simulink model "ALL_JP360_DBW_V6_5_1103"  (R2022a)
settings: Solver=FixedStepAuto  StartTime=0.0  StopTime=inf  FixedStep=0.01  RelTol=1e-3  EnableMultiTasking=on
model workspace (MAT data in the model file):
  g = 9.8
undefined symbols (not defined in the file or in its folder): canChannel, delta_v_p, IPM_Line_C0, IPM_Line_C1, IPM_Line_C2, IPM_Line_C3, M, M_p, MRR_ObjDistX, MRR_ObjDistY, MRR_ObjFusionCamID, MRR_ObjFusionSig, MRR_ObjID, MRR_ObjRelVelX, MRR_ObjRelVelY, MRR_ObjType, MRR_ObjUpdFlg, none, obj_vaild, untracktime, V, videoinput
libraries: canfdmsglib x230, canfdlib x76, slpidlib x24, simulink x18, dspstat3 x14, ctrlSharedLib x1, simulink_extras x1, imaqlib x1, realtime_pacer_lib x1, dspvision x1, visionsinks x1
(part 50 of 55)

== system ALL_JP360_DBW_V6_5_1103/button/ACCset/ACC_button ==
  Input : Inport
  SWM_ACCSwitch : Inport  Port=2
  SWM_ACCvSetPlus : Inport  Port=3
  SWM_ACCvSetMinus : Inport  Port=4
  set_speed_out : Inport  Port=5
  Add1 : Sum  Inputs=+-
  Add3 : Sum  Inputs=+-
  Add4 : Sum  Inputs=+-
  Chart1 : Stateflow chart  TreatAsAtomicUnit=on
      settings: RTWSystemCode=Reusable function
  Chart2 : Stateflow chart  TreatAsAtomicUnit=on
      settings: RTWSystemCode=Reusable function
  Data Store Read : DataStoreRead  DataStoreName=SpdSetValue  IndexOptions=Index vector (dialog)  Indices=1  OutputSizes=1
  Data Store Write2 : DataStoreWrite  DataStoreName=SpdSetValue  IndexOptions=Index vector (dialog)  Indices=1  OutputSizes=1
  Data Type Conversion : DataTypeConversion  OutDataTypeStr=uint8  SaturateOnIntegerOverflow=off  RndMeth=Floor
  Data Type Conversion1 : DataTypeConversion  OutDataTypeStr=single  SaturateOnIntegerOverflow=off  RndMeth=Floor
  Display : Display
  Memory{,1,7..8} (4 alike) : Memory
  OR3 : Logic  Operator=OR  Inputs=3  IconShape=distinctive  AllPortsSameDT=off  OutDataTypeStr=boolean
  Saturation : Saturate  UpperLimit=2  LowerLimit=0  OutDataTypeStr=int8
  Scope : Scope
  Subsystem1 : Subsystem  TreatAsAtomicUnit=on
      settings: MinAlgLoopOccurrences=on
  Subsystem2 : Subsystem  TreatAsAtomicUnit=on
      settings: MinAlgLoopOccurrences=on
  Subsystem3 : Subsystem  TreatAsAtomicUnit=on
      settings: MinAlgLoopOccurrences=on
  Subsystem4 : Subsystem  TreatAsAtomicUnit=on
      settings: MinAlgLoopOccurrences=on
  accsetv1 : Stateflow chart  TreatAsAtomicUnit=on
      settings: RTWSystemCode=Reusable function
  accsetv2 : Stateflow chart  TreatAsAtomicUnit=on
      settings: RTWSystemCode=Reusable function
  setvspeed : Outport
  SWM_ACCSwitchOut : Outport  Port=2
  wires:
  Subsystem3/1(Out1) -> Chart1/1(plus), Memory7/1, Add3/1
  Subsystem1/1(Out1) -> Memory8/1, Chart1/2(min), Add4/1
  [SWM_ACCvSetMinus] -> accsetv1/2(speed)
  SWM_ACCvSetPlus/1 -> [SWM_ACCvSetPlus]
  Memory7/1 -> Add3/2
  Chart1/1(a) -> Data Type Conversion/1, Display/1, Scope/1
  Add3/1 -> OR3/1
  SWM_ACCvSetMinus/1 -> [SWM_ACCvSetMinus]
  [SWM_ACCSwitch] -> Subsystem2/1(speedout)
  Input/1 -> [accsinp]
  Chart2/1(speedout) -> setvspeed/1
  SWM_ACCSwitch/1 -> [SWM_ACCSwitch]
  [SWM_ACCvSetPlus] -> accsetv2/2(speed)
  OR3/1 -> Chart1/Trigger
  Add4/1 -> OR3/2
  Memory8/1 -> Add4/2
  Subsystem2/1(Out1) -> Saturation/1
  Saturation/1 -> SWM_ACCSwitchOut/1  "SWM_ACCSwitchOut"
  [accstatus] -> accsetv1/1(accs)
  set_speed_out/1 -> Data Store Write2/1
  Memory1/1 -> Add1/2
  Data Store Read/1 -> Data Type Conversion1/1
  Add1/1 -> OR3/3
  [accsinp] -> Memory/1
  Memory/1 -> Subsystem4/1(speedout1)
  Subsystem4/1(Out1) -> [accstatus]
  accsetv2/1(speedout) -> Subsystem3/1(speedout)
  accsetv1/1(speedout) -> Subsystem1/1(speedout)
  [accstatus] -> accsetv2/1(accs)
  Data Type Conversion/1 -> Chart2/1(speed)
  Data Type Conversion1/1 -> Add1/1, Chart1/3(speed), Memory1/1

== system ALL_JP360_DBW_V6_5_1103/ACC_Control/ACC_FUNCTION/Subsystem2/ACC_model ==
  note: === Adaptive Cruise Control (ACC) autonomous system ===
      |
      |  - automatically controls the speed of the EGO vehicle,
      |  - is capable of assisting the driver to keep a safe distance
      |    from the preceding vehicle,
      |  - is controlling the engine throttle and brake pressure,
      |  - based on on-board, Technology Independent Sensors (TIS),
      |  - facilitates driving and partialy helps to prevent accidents.
  note: === ACC自适应巡航系统 ===
      |
      |  - 自动控制自车速度
      |  - 与前车保持安全距离
      |  - 自动控制刹车和油门防止碰撞
  note: 1/横摆角速度大于0.5°/s（可标定）时认为是过弯；
      | 2/弯道半径
  accstatus : Inport
  EGO_velocity_IC [m/s] : Inport  Port=2
  TIS1_range [m] : Inport  Port=3
  TIS1_rangedot [m/s] : Inport  Port=4
  HWT_dem [s] : Inport  Port=5
  Standstill_distance [m] : Inport  Port=6
  Des_speed[m/s] : Inport  Port=7
  obj_detacted_flag : Inport  Port=8
  abs_speed[m/s] : Inport  Port=9
  ax_esp[m/s2] : Inport  Port=10
  yaw_rate[deg/s] : Inport  Port=11
  steer_angle[deg] : Inport  Port=12
  ay_esp[m/s2] : Inport  Port=13
  IC_V_kph : Inport  Port=14
  CC_module : Subsystem  mask{DeltaV_Mul=5/3.6, Kp0=0.5, Kp1=0.01, Ki=0.005, Kd=0.05, Uplimit_acc=2, Uplimit_dec=-3}
      mask prompts: DeltaV_Mul "速度分段控制DeltaV_Mul"; Kp0 "速度误差大时Kp0"; Kp1 "速度误差小时Kp1"; Ki "定速巡航KI"; Kd "定速巡航Kd"; Uplimit_acc "定速巡航加速度上限Uplimit_acc"; Uplimit_dec "定速巡航减速度上线Uplimit_dec"
      mask DialogControl ParameterGroupVar Prompt: 参数
  Constant : Constant  Value=0  OutDataTypeStr=single
  Dead Zone : DeadZone  LowerValue=-1.2/57.3  UpperValue=1.2/57.3
  Gain3 : Gain  Gain=1/57.3
  Product : Product
  Rate transition from other signals1 : Subsystem  Commented=on
  Rate transition from EGO1 : Subsystem  Commented=on
  Rate transition from TIS2 : Subsystem  Commented=on
  Saturation1 : Saturate  UpperLimit=20/57.3  LowerLimit=-20/57.3
  Scope : Scope  NumInputPorts=2
  TIS1 ACC action : Subsystem
  calculate_slope : Subsystem
  curve agl : Subsystem
  acc_acceleration [a] : Outport
  acc_deceleration [-a] : Outport  Port=2
  MODE_OUT : Outport  Port=3
  slope : Outport  Port=4
  standstill_req : Outport  Port=5  InitialOutput=[150]
  wires:
  TIS1 ACC action/1(acceleration[a]) -> Scope/1, acc_acceleration [a]/1
  Dead Zone/1 -> Saturation1/1
  IC_V_kph/1 -> CC_module/3(IC_V_kph)
  [Des_speed] -> curve agl/3(desire_speed)
  TIS1 ACC action/2(deceleration[-a]) -> Scope/2, acc_deceleration [-a]/1
  [ay_esp] -> curve agl/2(ay_esp)
  curve agl/1(Output) -> [Ded_speed_2]
  [EGO_velocity] -> TIS1 ACC action/1(v_ego)
  Des_speed[m/s]/1 -> [Des_speed]
  steer_angle[deg]/1 -> [steer_angle]
  [cc_acceleration_in] -> TIS1 ACC action/4(cc_acceleration_in)
  [abs_speed] -> calculate_slope/4(vx1)
  obj_detacted_flag/1 -> TIS1 ACC action/9(obj_detacted_flag)
  [yaw_rate] -> Gain3/1
  TIS1_range [m]/1 -> [TIS1_range]
  [TIS1_range] -> TIS1 ACC action/3(d_obj)
  ax_esp[m/s2]/1 -> [ax_esp]
  [TIS1_rangedot] -> TIS1 ACC action/2(v_obj)
  [Standstill] -> TIS1 ACC action/8(standstill)
  TIS1 ACC action/3(ACC_MODE) -> MODE_OUT/1
  [Ded_speed_2] -> CC_module/2(Desired Velocity [m/s]), TIS1 ACC action/6(v_set)
  [cc_deceleration_in] -> TIS1 ACC action/5(cc_deceleration_in)
  [steer_angle] -> calculate_slope/3(δ)
  [ax_esp] -> calculate_slope/1(ax_esp)
  Standstill_distance [m]/1 -> [Standstill]
  TIS1_rangedot [m/s]/1 -> [TIS1_rangedot]
  CC_module/1(cc_acceleration [a]) -> [cc_acceleration_in]
  HWT_dem [s]/1 -> [HWT_dem]
  [abs_speed] -> CC_module/1(velocity [m/s])
  [HWT_dem] -> TIS1 ACC action/7(t_dem)
  calculate_slope/1(φ) -> Dead Zone/1
  EGO_velocity_IC [m/s]/1 -> [EGO_velocity]
  Product/1 -> slope/1
  abs_speed[m/s]/1 -> [abs_speed]
  TIS1 ACC action/4(standstill_req) -> standstill_req/1
  ay_esp[m/s2]/1 -> [ay_esp]
  yaw_rate[deg/s]/1 -> [yaw_rate]
  Gain3/1 -> calculate_slope/2(ω)
  [yaw_rate] -> curve agl/1(yaw_rate)
  CC_module/2(cc_deceleration [-a]) -> [cc_deceleration_in]
  accstatus/1 -> [accstatus]
  [accstatus] -> CC_module/4(ACC_STATUSt)
  Saturation1/1 -> Product/1
  Constant/1 -> Product/2

== system ALL_JP360_DBW_V6_5_1103/ACC_Control/ACC_FUNCTION/Subsystem2/Limit ==
  note: 油门减速度互斥
  note: 对减速度斜率进行限幅
      | 1，减速度<-0.6，减速度斜率上升沿为0.13，下降沿为0.6；
      | 2，减速度>-0.6，减速度斜率上升沿为0.13，下降沿为0.17.
  note: 对加速度进行限幅
      | 1，速度>60kph，加速度最大为1.5；
      | 2，速度<60kph，加速度最大为0.6
  acc[a] : Inport
  dec[-a] : Inport  Port=2
  slope : Inport  Port=3
  Set_speed_mps : Inport  Port=4
  IC_V_kph : Inport  Port=5
  ACC_MODE : Inport  Port=6
  IC_V_mps : Inport  Port=7
  abs_mps : Inport  Port=8
  ACC_STATUS : Inport  Port=9
  delta_v : Inport  Port=10
  Add : Sum  Inputs=+-
  Add1 : Sum  Commented=on  Inputs=-+
  Add2 : Sum
  Chart1 : Stateflow chart  TreatAsAtomicUnit=on
      settings: PortSchema="{\"entries\":[{\"content\":{\"sides\":[{\"content\":{\"connectorIds\":[\"In1\",\"In3\",\"In2\",\"In4\"]},\"type\":\"ConnectorPlacement.EquallySpacedRectSide\",\"uuid\":\"a1ea63d3-d60a-460d-bbc1-1bfef8c0288a\"},{\"content\":{\"connectorIds\":[\"Out1\",\"Out2\"],\"side\":\"RIGHT\"},\"type\":\"ConnectorPlacement.EquallySpacedRectSide\",\"uuid\":\"c1973d49-ef12-4d82-bde3-89be47febb9b\"},{\"content\":{\"connectorIds\":[],\"side\":\"TOP\"},\"type\":\"ConnectorPlacement.EquallySpacedRectSide\",\"uuid\":\"7d8c7564-58f8-4cff-9ab8-be78f521a8c3\"}]},\"type\":\"ConnectorPlacement.EquallySpacedConnector\",\"uuid\":\"5e34bcad-cbf5-413a-b462-ddd7cae783c7\"}],\"packageUris\":[\"http://schema.mathworks.com/mf0/Connector/R2020b\"],\"version\":\"1.0\"}"
  Constant1 : Constant  Value=6  OutDataTypeStr=int8
  Constant3 : Constant  Value=-10  OutDataTypeStr=single
  Dead Zone : DeadZone  LowerValue=-0.05  UpperValue=0
  From10 : From  Commented=on  GotoTag=abs_kph
  From11 : From  Commented=on  GotoTag=Set_speed_mps
  From12 : From  Commented=on  GotoTag=decout
  Gain : Gain  Commented=on  Gain=3.6
  Goto8 : Goto  Commented=on  GotoTag=decin
  MATLAB Function : MATLAB Function  Commented=on  TreatAsAtomicUnit=on
  Memory : Memory
  Mux : Mux  Inputs=2
  Rate Limiter1 : RateLimiter  RisingSlewLimit=1000  SampleTimeMode=inherited
  Rate Limiter2 : RateLimiter  Commented=through  RisingSlewLimit=0.5  FallingSlewLimit=-0.3  SampleTimeMode=inherited
  Rate Limiter3 : RateLimiter  Commented=through  RisingSlewLimit=0.5  FallingSlewLimit=-0.1  SampleTimeMode=inherited
  Rate Limiter4 : RateLimiter  RisingSlewLimit=1000  SampleTimeMode=inherited
  Saturation : Saturate  Commented=through  UpperLimit=Uplimit_a  LowerLimit=0
  Saturation1 : Saturate  Commented=through  UpperLimit=Lowlimit_a  LowerLimit=0
  Saturation2 : Saturate  UpperLimit=1000000  LowerLimit=-10
  Scope : Scope  NumInputPorts=4
  Scope1 : Scope  NumInputPorts=2
  Switch1 : Switch  Criteria=u2 ~= 0  SaturateOnIntegerOverflow=off  InputSameDT=off
  Switch2 : Switch  Criteria=u2 > Threshold  Threshold=V_limit_line  SaturateOnIntegerOverflow=off  InputSameDT=off
  Switch3 : Switch  Threshold=-20  SaturateOnIntegerOverflow=off  InputSameDT=off
  a2m_表达式 : Subsystem  Commented=on
  a2m_表达式_标定表 : Subsystem
  acceleration_throttle——PID : Subsystem  Commented=on
  brake_deadzone : Constant  Value=Dec_dead_zone  OutDataTypeStr=single
  a&-a : Outport
  M_slope : Outport  Port=2
  M_a : Outport  Port=3
  M_cc : Outport  Port=4
  M_pid : Outport  Port=5
  wires:
  a2m_表达式_标定表/5(M_pid) -> M_pid/1
  a2m_表达式_标定表/4(M_cc) -> M_cc/1
  a2m_表达式_标定表/3(M_a) -> M_a/1
  a2m_表达式_标定表/2(M_slope) -> M_slope/1
  IC_V_mps/1 -> [Ic_v_mps]
  [Ic_v_kph] -> a2m_表达式_标定表/2(IC_V_kph)
  [acc] -> Saturation/1, Saturation1/1
  Set_speed_mps/1 -> [Set_speed_mps]
  slope/1 -> a2m_表达式_标定表/3(slope)
  Add2/1 -> Chart1/1(acc), Scope1/2
  [dec] -> Dead Zone/1
  [Set_speed_mps] -> a2m_表达式_标定表/5(Set_speed_mps1)
  Add/1 -> Switch1/2
  ACC_MODE/1 -> Add/1
  Constant1/1 -> Add/2
  [decout] -> Scope/3  "dec"
  [acc] -> Scope/2
  [Ic_v_kph] -> Scope/1
  Switch1/1 -> [decout], Scope1/1  "dec_out"
  Dead Zone/1 -> Rate Limiter3/1, Rate Limiter2/1, Switch1/3
  IC_V_kph/1 -> [Ic_v_kph]
  [Ego_velocity_abs_kph] -> Switch2/2
  Mux/1 -> a&-a/1
  dec[-a]/1 -> [dec]
  Saturation1/1 -> Switch2/3
  acc[a]/1 -> [acc]  "a_in"
  Saturation/1 -> Switch2/1
  Switch2/1 -> a2m_表达式/2(acce), acceleration_throttle——PID/3(acce1), a2m_表达式_标定表/1(acce)
  brake_deadzone/1 -> Chart1/2(brake_kt)
  Chart1/1(trottle) -> Mux/1, Scope/4  "torqur_out"
  abs_mps/1 -> [abs_mps]
  [abs_mps] -> a2m_表达式_标定表/6(abs_mps1)
  ACC_STATUS/1 -> [ACC_STATUS]
  [ACC_STATUS] -> a2m_表达式_标定表/4(ACC_STATUSt)
  From10/1 -> Add1/1
  From11/1 -> Gain/1
  Add1/1 -> MATLAB Function/1(u)
  a2m_表达式_标定表/1(throttle[NM]) -> Saturation2/1
  MATLAB Function/1(y1) -> Add2/1
  From12/1 -> MATLAB Function/2(data)
  MATLAB Function/2(y2) -> Goto8/1
  [decout] -> Chart1/3(dec)
  Gain/1 -> Add1/2
  Constant3/1 -> Chart1/4(t)
  Chart1/2(brake) -> [dec_m], Mux/2
  [dec_m] -> Memory/1
  Memory/1 -> a2m_表达式_标定表/7(dec_m)
  Rate Limiter3/1 -> Rate Limiter1/1
  Rate Limiter2/1 -> Rate Limiter4/1
  delta_v/1 -> Switch3/2
  Switch3/1 -> Switch1/1
  Rate Limiter1/1 -> Switch3/1
  Rate Limiter4/1 -> Switch3/3
  Saturation2/1 -> Add2/2

== system ALL_JP360_DBW_V6_5_1103/ACC_Control/ACC_FUNCTION/Subsystem2/override ==
  In1 : Inport
  In2 : Inport  Port=2
  In3 : Inport  Port=3
  In4 : Inport  Port=4
  Abs1 : Abs  SaturateOnIntegerOverflow=off
  Abs2 : Abs  SaturateOnIntegerOverflow=off
  Add{1,3,7..8} (4 alike) : Sum  Inputs=+-
  Chart2 : Stateflow chart  TreatAsAtomicUnit=on
  Constant12 : Constant  Value=15  OutDataTypeStr=single
  Constant17 : Constant  Value=2  OutDataTypeStr=single
  Constant7 : Constant  Value=2.5  OutDataTypeStr=single
  Data Store Read : DataStoreRead  DataStoreName=acc_change_mode  IndexOptions=Index vector (dialog)  Indices=1  OutputSizes=1
  Data Store Write1 : DataStoreWrite  DataStoreName=acc_change_mode  IndexOptions=Index vector (dialog)  Indices=1  OutputSizes=1
  Data Store Write2 : DataStoreWrite  DataStoreName=acc_change_mode  IndexOptions=Index vector (dialog)  Indices=1  OutputSizes=1
  Data Store Write3 : DataStoreWrite  DataStoreName=acc_change_mode  IndexOptions=Index vector (dialog)  Indices=1  OutputSizes=1
  Data Type Conversion{,1..2,7} (4 alike) : DataTypeConversion  OutDataTypeStr=single  SaturateOnIntegerOverflow=off  RndMeth=Floor
  Memory1 : Memory
  Memory2 : Memory
  Memory3 : Memory
  Mux2 : Mux  Inputs=2
  Product : Product
  Product3 : Product
  Relational Operator : RelationalOperator  Operator=<=  OutDataTypeStr=boolean  RndMeth=Simplest  InputSameDT=off
  Relational Operator1 : RelationalOperator  Operator===  OutDataTypeStr=boolean  RndMeth=Simplest  InputSameDT=off
  Relational Operator3 : RelationalOperator  Operator===  OutDataTypeStr=boolean  RndMeth=Simplest  InputSameDT=off
  Saturation1 : Saturate  UpperLimit=1  LowerLimit=0
  Saturation2 : Saturate  UpperLimit=1  LowerLimit=0
  override_mode : Outport
  wires:
  Abs1/1 -> Saturation1/1
  Mux2/1 -> Chart2/Trigger
  Saturation1/1 -> Data Type Conversion/1
  Memory1/1 -> Add7/2
  In4/1 -> Add8/2, Product/1, Memory2/1
  Data Type Conversion7/1 -> Mux2/1
  In1/1 -> Add7/1, Memory1/1
  Relational Operator/1 -> Data Type Conversion1/1
  Add7/1 -> Abs1/1
  Add3/1 -> Relational Operator/1
  Constant7/1 -> Relational Operator/2
  Relational Operator3/1 -> Product3/2
  Relational Operator1/1 -> Product3/1
  Constant17/1 -> Relational Operator3/1
  Constant12/1 -> Relational Operator1/1
  Memory2/1 -> Add8/1, Product/2
  Add8/1 -> Relational Operator3/2
  Product/1 -> Relational Operator1/2
  Product3/1 -> Data Type Conversion7/1
  Data Store Read/1 -> Mux2/2
  In2/1 -> Add3/1
  Chart2/1(u1) -> override_mode/1
  Data Type Conversion/1 -> Data Store Write2/1
  Data Type Conversion1/1 -> Data Store Write1/1
  Memory3/1 -> Add1/2
  Data Type Conversion2/1 -> Data Store Write3/1
  Abs2/1 -> Saturation2/1
  In3/1 -> Add1/1, Memory3/1, Add3/2
  Saturation2/1 -> Data Type Conversion2/1
  Add1/1 -> Abs2/1

== system ALL_JP360_DBW_V6_5_1103/CIPV1/Obstacle selection/Subsystem/Subsystem ==
  MRR_ObjID : Inport
  MRR_ObjDistX : Inport  Port=2
  MRR_ObjDistY : Inport  Port=3
  MRR_ObjRelVelX : Inport  Port=4
  MRR_ObjRelVelY : Inport  Port=5
  MRR_ObjType : Inport  Port=6
  CIPV_index1 : Inport  Port=7
  MRR_ObjUpdFlg : Inport  Port=8
  obj_vaild : Inport  Port=9
  IPM_obj : Inport  Port=10
  MRR_ObjFusionSig : Inport  Port=11
  MRR_ObjFusionCamID : Inport  Port=12
  Bus Creator1 : BusCreator  Inputs=MRR_ObjID,MRR_ObjDistX,MRR_ObjDistY,MRR_ObjRelVelX,MRR_ObjRelVelY,MRR_ObjType,MRR_ObjUpdFlg,obj_vaild,untracktime,MRR_ObjFusionCamID,MRR_ObjFusionSig
  Bus Creator2 : BusCreator  Inputs=MRR_ObjID,MRR_ObjDistX,MRR_ObjDistY,MRR_ObjRelVelX,MRR_ObjRelVelY,MRR_ObjType,MRR_ObjUpdFlg,obj_vaild,untracktime,MRR_ObjFusionCamID,MRR_ObjFusionSig
  Constant{,2..8,10..12} (11 alike) : Constant  Value=0  OutDataTypeStr=single
  Constant1 : Constant  Value=[0 0 0 0 0 3 2 1]  OutDataTypeStr=single
  Constant9 : Constant  Value=0  OutDataTypeStr=uint8
  MATLAB Function : MATLAB Function  TreatAsAtomicUnit=on
  Selector{,1..6,8..11} (11 alike) : Selector  InputPortWidth=32  IndexOptions=Index vector (port)  Indices=[1 3]  OutputSizes=1
  Selector7 : Selector  IndexMode=Zero-based  InputPortWidth=8  IndexOptions=Index vector (port)  Indices=[1 3]  OutputSizes=1
  Switch4 : Switch  Criteria=u2 > Threshold  SaturateOnIntegerOverflow=off  InputSameDT=off
  cipv1 : Outport
  wires:
  Bus Creator1/1 -> Switch4/1
  CIPV_index1/1 -> [CIPV_index1]
  MRR_ObjID/1 -> Selector/1
  [CIPV_index1] -> Selector/2
  Selector/1 -> Bus Creator1/1  "MRR_ObjID"
  MRR_ObjDistX/1 -> Selector1/1
  [CIPV_index1] -> Selector1/2
  Selector1/1 -> Bus Creator1/2  "MRR_ObjDistX"
  MRR_ObjDistY/1 -> Selector2/1
  [CIPV_index1] -> Selector2/2
  Selector2/1 -> Bus Creator1/3  "MRR_ObjDistY"
  MRR_ObjRelVelX/1 -> Selector3/1
  [CIPV_index1] -> Selector3/2
  Selector3/1 -> Bus Creator1/4  "MRR_ObjRelVelX"
  MRR_ObjRelVelY/1 -> Selector4/1
  [CIPV_index1] -> Selector4/2
  Selector4/1 -> Bus Creator1/5  "MRR_ObjRelVelY"
  [CIPV_index1] -> Selector5/2
  [obj_vaild] -> Bus Creator1/8  "obj_vaild"
  Constant/1 -> Bus Creator1/9  "untracktime"
  [CIPV_index1] -> Selector6/2
  MRR_ObjUpdFlg/1 -> Selector6/1
  Selector6/1 -> Bus Creator1/7  "MRR_ObjUpdFlg"
  Constant1/1 -> Selector7/1
  Selector7/1 -> Bus Creator1/6  "MRR_ObjType"
  obj_vaild/1 -> [obj_vaild]  "obj_vaild"
  [obj_vaild] -> Switch4/2
  Bus Creator2/1 -> Switch4/3
  Switch4/1 -> cipv1/1
  Constant3/1 -> Bus Creator2/1  "MRR_ObjID"
  Constant2/1 -> Bus Creator2/2  "MRR_ObjDistX"
  Constant4/1 -> Bus Creator2/3  "MRR_ObjDistY"
  Constant5/1 -> Bus Creator2/4  "MRR_ObjRelVelX"
  Constant6/1 -> Bus Creator2/5  "MRR_ObjRelVelY"
  Constant7/1 -> Bus Creator2/6  "MRR_ObjType"
  Constant8/1 -> Bus Creator2/7  "MRR_ObjUpdFlg"
  Constant9/1 -> Bus Creator2/8  "obj_vaild"
  Constant10/1 -> Bus Creator2/9  "untracktime"
  IPM_obj/1 -> [IPM_obj]
  MRR_ObjFusionSig/1 -> [MRR_ObjFusionSig]
  MRR_ObjFusionCamID/1 -> [MRR_ObjFusionCamID]
  MRR_ObjType/1 -> [MRR_ObjType]
  [MRR_ObjType] -> Selector5/1
  MATLAB Function/1(y) -> Selector7/2
  Selector5/1 -> MATLAB Function/1(mrr_type)
  Selector10/1 -> MATLAB Function/4(hasCamera)
  [MRR_ObjFusionSig] -> Selector10/1
  [CIPV_index1] -> Selector8/2
  [CIPV_index1] -> Selector10/2
  Selector8/1 -> MATLAB Function/2(ipm_id)
  [MRR_ObjFusionCamID] -> Selector8/1
  [IPM_obj] -> MATLAB Function/3(ipm_obj)
  [MRR_ObjFusionCamID] -> Selector9/1
  [CIPV_index1] -> Selector9/2
  Selector9/1 -> Bus Creator1/10  "MRR_ObjFusionCamID"
  [CIPV_index1] -> Selector11/2
  [MRR_ObjFusionSig] -> Selector11/1
  Selector11/1 -> Bus Creator1/11  "MRR_ObjFusionSig"
  Constant11/1 -> Bus Creator2/10  "MRR_ObjFusionCamID"
  Constant12/1 -> Bus Creator2/11  "MRR_ObjFusionSig"

== system ALL_JP360_DBW_V6_5_1103/CIPV1/Obstacle selection/Subsystem/Subsystem1 ==
  MRR_ObjID : Inport
  MRR_ObjDistX : Inport  Port=2
  MRR_ObjDistY : Inport  Port=3
  MRR_ObjRelVelX : Inport  Port=4
  MRR_ObjRelVelY : Inport  Port=5
  MRR_ObjType : Inport  Port=6
  CIPV_index1 : Inport  Port=7
  MRR_ObjUpdFlg : Inport  Port=8
  obj_vaild : Inport  Port=9
  IPM_obj : Inport  Port=10
  MRR_ObjFusionSig : Inport  Port=11
  MRR_ObjFusionCamID : Inport  Port=12
  Bus Creator1 : BusCreator  Inputs=MRR_ObjID,MRR_ObjDistX,MRR_ObjDistY,MRR_ObjRelVelX,MRR_ObjRelVelY,MRR_ObjType,MRR_ObjUpdFlg,obj_vaild,untracktime,MRR_ObjFusionCamID,MRR_ObjFusionSig
  Bus Creator2 : BusCreator  Inputs=MRR_ObjID,MRR_ObjDistX,MRR_ObjDistY,MRR_ObjRelVelX,MRR_ObjRelVelY,MRR_ObjType,MRR_ObjUpdFlg,obj_vaild,untracktime,MRR_ObjFusionCamID,MRR_ObjFusionSig
  Constant{,2..8,10..12} (11 alike) : Constant  Value=0  OutDataTypeStr=single
  Constant1 : Constant  Value=[0 0 0 0 0 3 2 1]  OutDataTypeStr=single
  Constant9 : Constant  Value=0  OutDataTypeStr=uint8
  MATLAB Function : MATLAB Function  TreatAsAtomicUnit=on
  Selector{,1..6,8..11} (11 alike) : Selector  InputPortWidth=32  IndexOptions=Index vector (port)  Indices=[1 3]  OutputSizes=1
  Selector7 : Selector  IndexMode=Zero-based  InputPortWidth=8  IndexOptions=Index vector (port)  Indices=[1 3]  OutputSizes=1
  Switch4 : Switch  Criteria=u2 > Threshold  SaturateOnIntegerOverflow=off  InputSameDT=off
  cipv1 : Outport
  wires:
  Constant12/1 -> Bus Creator2/11  "MRR_ObjFusionSig"
  Constant11/1 -> Bus Creator2/10  "MRR_ObjFusionCamID"
  Selector11/1 -> Bus Creator1/11  "MRR_ObjFusionSig"
  [MRR_ObjFusionSig] -> Selector11/1
  [CIPV_index1] -> Selector11/2
  Selector9/1 -> Bus Creator1/10  "MRR_ObjFusionCamID"
  [CIPV_index1] -> Selector9/2
  [MRR_ObjFusionCamID] -> Selector9/1
  [IPM_obj] -> MATLAB Function/3(ipm_obj)
  [MRR_ObjFusionCamID] -> Selector8/1
  Selector8/1 -> MATLAB Function/2(ipm_id)
  [CIPV_index1] -> Selector10/2
  [CIPV_index1] -> Selector8/2
  [MRR_ObjFusionSig] -> Selector10/1
  Selector10/1 -> MATLAB Function/4(hasCamera)
  Selector5/1 -> MATLAB Function/1(mrr_type)
  MATLAB Function/1(y) -> Selector7/2
  [MRR_ObjType] -> Selector5/1
  MRR_ObjType/1 -> [MRR_ObjType]
  MRR_ObjFusionCamID/1 -> [MRR_ObjFusionCamID]
  MRR_ObjFusionSig/1 -> [MRR_ObjFusionSig]
  IPM_obj/1 -> [IPM_obj]
  Constant10/1 -> Bus Creator2/9  "untracktime"
  Constant9/1 -> Bus Creator2/8  "obj_vaild"
  Constant8/1 -> Bus Creator2/7  "MRR_ObjUpdFlg"
  Constant7/1 -> Bus Creator2/6  "MRR_ObjType"
  Constant6/1 -> Bus Creator2/5  "MRR_ObjRelVelY"
  Constant5/1 -> Bus Creator2/4  "MRR_ObjRelVelX"
  Constant4/1 -> Bus Creator2/3  "MRR_ObjDistY"
  Constant2/1 -> Bus Creator2/2  "MRR_ObjDistX"
  Constant3/1 -> Bus Creator2/1  "MRR_ObjID"
  Switch4/1 -> cipv1/1
  Bus Creator2/1 -> Switch4/3
  [obj_vaild] -> Switch4/2
  obj_vaild/1 -> [obj_vaild]  "obj_vaild"
  Selector7/1 -> Bus Creator1/6  "MRR_ObjType"
  Constant1/1 -> Selector7/1
  Selector6/1 -> Bus Creator1/7  "MRR_ObjUpdFlg"
  MRR_ObjUpdFlg/1 -> Selector6/1
  [CIPV_index1] -> Selector6/2
  Constant/1 -> Bus Creator1/9  "untracktime"
  [obj_vaild] -> Bus Creator1/8  "obj_vaild"
  [CIPV_index1] -> Selector5/2
  Selector4/1 -> Bus Creator1/5  "MRR_ObjRelVelY"
  [CIPV_index1] -> Selector4/2
  MRR_ObjRelVelY/1 -> Selector4/1
  Selector3/1 -> Bus Creator1/4  "MRR_ObjRelVelX"
  [CIPV_index1] -> Selector3/2
  MRR_ObjRelVelX/1 -> Selector3/1
  Selector2/1 -> Bus Creator1/3  "MRR_ObjDistY"
  [CIPV_index1] -> Selector2/2
  MRR_ObjDistY/1 -> Selector2/1
  Selector1/1 -> Bus Creator1/2  "MRR_ObjDistX"
  [CIPV_index1] -> Selector1/2
  MRR_ObjDistX/1 -> Selector1/1
  Selector/1 -> Bus Creator1/1  "MRR_ObjID"
  [CIPV_index1] -> Selector/2
  MRR_ObjID/1 -> Selector/1
  CIPV_index1/1 -> [CIPV_index1]
  Bus Creator1/1 -> Switch4/1

== system ALL_JP360_DBW_V6_5_1103/CIPV1/Obstacle selection/Subsystem/Subsystem2 ==
  MRR_ObjID : Inport
  MRR_ObjDistX : Inport  Port=2
  MRR_ObjDistY : Inport  Port=3
  MRR_ObjRelVelX : Inport  Port=4
  MRR_ObjRelVelY : Inport  Port=5
  MRR_ObjType : Inport  Port=6
  CIPV_index1 : Inport  Port=7
  MRR_ObjUpdFlg : Inport  Port=8
  obj_vaild : Inport  Port=9
  IPM_obj : Inport  Port=10
  MRR_ObjFusionSig : Inport  Port=11
  MRR_ObjFusionCamID : Inport  Port=12
  Bus Creator1 : BusCreator  Inputs=MRR_ObjID,MRR_ObjDistX,MRR_ObjDistY,MRR_ObjRelVelX,MRR_ObjRelVelY,MRR_ObjType,MRR_ObjUpdFlg,obj_vaild,untracktime,MRR_ObjFusionCamID,MRR_ObjFusionSig
  Bus Creator2 : BusCreator  Inputs=MRR_ObjID,MRR_ObjDistX,MRR_ObjDistY,MRR_ObjRelVelX,MRR_ObjRelVelY,MRR_ObjType,MRR_ObjUpdFlg,obj_vaild,untracktime,MRR_ObjFusionCamID,MRR_ObjFusionSig
  Constant{,2..8,10..12} (11 alike) : Constant  Value=0  OutDataTypeStr=single
  Constant1 : Constant  Value=[0 0 0 0 0 3 2 1]  OutDataTypeStr=single
  Constant9 : Constant  Value=0  OutDataTypeStr=uint8
  MATLAB Function : MATLAB Function  TreatAsAtomicUnit=on
  Selector{,1..6,8..11} (11 alike) : Selector  InputPortWidth=32  IndexOptions=Index vector (port)  Indices=[1 3]  OutputSizes=1
  Selector7 : Selector  IndexMode=Zero-based  InputPortWidth=8  IndexOptions=Index vector (port)  Indices=[1 3]  OutputSizes=1
  Switch4 : Switch  Criteria=u2 > Threshold  SaturateOnIntegerOverflow=off  InputSameDT=off
  cipv1 : Outport
  wires:
  Bus Creator1/1 -> Switch4/1
  CIPV_index1/1 -> [CIPV_index1]
  MRR_ObjID/1 -> Selector/1
  [CIPV_index1] -> Selector/2
  Selector/1 -> Bus Creator1/1  "MRR_ObjID"
  MRR_ObjDistX/1 -> Selector1/1
  [CIPV_index1] -> Selector1/2
  Selector1/1 -> Bus Creator1/2  "MRR_ObjDistX"
  MRR_ObjDistY/1 -> Selector2/1
  [CIPV_index1] -> Selector2/2
  Selector2/1 -> Bus Creator1/3  "MRR_ObjDistY"
  MRR_ObjRelVelX/1 -> Selector3/1
  [CIPV_index1] -> Selector3/2
  Selector3/1 -> Bus Creator1/4  "MRR_ObjRelVelX"
  MRR_ObjRelVelY/1 -> Selector4/1
  [CIPV_index1] -> Selector4/2
  Selector4/1 -> Bus Creator1/5  "MRR_ObjRelVelY"
  [CIPV_index1] -> Selector5/2
  [obj_vaild] -> Bus Creator1/8  "obj_vaild"
  Constant/1 -> Bus Creator1/9  "untracktime"
  [CIPV_index1] -> Selector6/2
  MRR_ObjUpdFlg/1 -> Selector6/1
  Selector6/1 -> Bus Creator1/7  "MRR_ObjUpdFlg"
  Constant1/1 -> Selector7/1
  Selector7/1 -> Bus Creator1/6  "MRR_ObjType"
  obj_vaild/1 -> [obj_vaild]  "obj_vaild"
  [obj_vaild] -> Switch4/2
  Bus Creator2/1 -> Switch4/3
  Switch4/1 -> cipv1/1
  Constant3/1 -> Bus Creator2/1  "MRR_ObjID"
  Constant2/1 -> Bus Creator2/2  "MRR_ObjDistX"
  Constant4/1 -> Bus Creator2/3  "MRR_ObjDistY"
  Constant5/1 -> Bus Creator2/4  "MRR_ObjRelVelX"
  Constant6/1 -> Bus Creator2/5  "MRR_ObjRelVelY"
  Constant7/1 -> Bus Creator2/6  "MRR_ObjType"
  Constant8/1 -> Bus Creator2/7  "MRR_ObjUpdFlg"
  Constant9/1 -> Bus Creator2/8  "obj_vaild"
  Constant10/1 -> Bus Creator2/9  "untracktime"
  IPM_obj/1 -> [IPM_obj]
  MRR_ObjFusionSig/1 -> [MRR_ObjFusionSig]
  MRR_ObjFusionCamID/1 -> [MRR_ObjFusionCamID]
  MRR_ObjType/1 -> [MRR_ObjType]
  [MRR_ObjType] -> Selector5/1
  MATLAB Function/1(y) -> Selector7/2
  Selector5/1 -> MATLAB Function/1(mrr_type)
  Selector10/1 -> MATLAB Function/4(hasCamera)
  [MRR_ObjFusionSig] -> Selector10/1
  [CIPV_index1] -> Selector8/2
  [CIPV_index1] -> Selector10/2
  Selector8/1 -> MATLAB Function/2(ipm_id)
  [MRR_ObjFusionCamID] -> Selector8/1
  [IPM_obj] -> MATLAB Function/3(ipm_obj)
  [MRR_ObjFusionCamID] -> Selector9/1
  [CIPV_index1] -> Selector9/2
  Selector9/1 -> Bus Creator1/10  "MRR_ObjFusionCamID"
  [CIPV_index1] -> Selector11/2
  [MRR_ObjFusionSig] -> Selector11/1
  Selector11/1 -> Bus Creator1/11  "MRR_ObjFusionSig"
  Constant11/1 -> Bus Creator2/10  "MRR_ObjFusionCamID"
  Constant12/1 -> Bus Creator2/11  "MRR_ObjFusionSig"

== system ALL_JP360_DBW_V6_5_1103/CIPV1/Obstacle selection/Subsystem/Subsystem3 ==
  MRR_ObjID : Inport
  MRR_ObjDistX : Inport  Port=2
  MRR_ObjDistY : Inport  Port=3
  MRR_ObjRelVelX : Inport  Port=4
  MRR_ObjRelVelY : Inport  Port=5
  MRR_ObjType : Inport  Port=6
  CIPV_index1 : Inport  Port=7
  MRR_ObjUpdFlg : Inport  Port=8
  obj_vaild : Inport  Port=9
  IPM_obj : Inport  Port=10
  MRR_ObjFusionSig : Inport  Port=11
  MRR_ObjFusionCamID : Inport  Port=12
  Bus Creator1 : BusCreator  Inputs=MRR_ObjID,MRR_ObjDistX,MRR_ObjDistY,MRR_ObjRelVelX,MRR_ObjRelVelY,MRR_ObjType,MRR_ObjUpdFlg,obj_vaild,untracktime,MRR_ObjFusionCamID,MRR_ObjFusionSig
  Bus Creator2 : BusCreator  Inputs=MRR_ObjID,MRR_ObjDistX,MRR_ObjDistY,MRR_ObjRelVelX,MRR_ObjRelVelY,MRR_ObjType,MRR_ObjUpdFlg,obj_vaild,untracktime,MRR_ObjFusionCamID,MRR_ObjFusionSig
  Constant{,2..8,10..12} (11 alike) : Constant  Value=0  OutDataTypeStr=single
  Constant1 : Constant  Value=[0 0 0 0 0 3 2 1]  OutDataTypeStr=single
  Constant9 : Constant  Value=0  OutDataTypeStr=uint8
  MATLAB Function : MATLAB Function  TreatAsAtomicUnit=on
  Selector{,1..6,8..11} (11 alike) : Selector  InputPortWidth=32  IndexOptions=Index vector (port)  Indices=[1 3]  OutputSizes=1
  Selector7 : Selector  IndexMode=Zero-based  InputPortWidth=8  IndexOptions=Index vector (port)  Indices=[1 3]  OutputSizes=1
  Switch4 : Switch  Criteria=u2 > Threshold  SaturateOnIntegerOverflow=off  InputSameDT=off
  cipv1 : Outport
  wires:
  Bus Creator1/1 -> Switch4/1
  CIPV_index1/1 -> [CIPV_index1]
  MRR_ObjID/1 -> Selector/1
  [CIPV_index1] -> Selector/2
  Selector/1 -> Bus Creator1/1  "MRR_ObjID"
  MRR_ObjDistX/1 -> Selector1/1
  [CIPV_index1] -> Selector1/2
  Selector1/1 -> Bus Creator1/2  "MRR_ObjDistX"
  MRR_ObjDistY/1 -> Selector2/1
  [CIPV_index1] -> Selector2/2
  Selector2/1 -> Bus Creator1/3  "MRR_ObjDistY"
  MRR_ObjRelVelX/1 -> Selector3/1
  [CIPV_index1] -> Selector3/2
  Selector3/1 -> Bus Creator1/4  "MRR_ObjRelVelX"
  MRR_ObjRelVelY/1 -> Selector4/1
  [CIPV_index1] -> Selector4/2
  Selector4/1 -> Bus Creator1/5  "MRR_ObjRelVelY"
  [CIPV_index1] -> Selector5/2
  [obj_vaild] -> Bus Creator1/8  "obj_vaild"
  Constant/1 -> Bus Creator1/9  "untracktime"
  [CIPV_index1] -> Selector6/2
  MRR_ObjUpdFlg/1 -> Selector6/1
  Selector6/1 -> Bus Creator1/7  "MRR_ObjUpdFlg"
  Constant1/1 -> Selector7/1
  Selector7/1 -> Bus Creator1/6  "MRR_ObjType"
  obj_vaild/1 -> [obj_vaild]  "obj_vaild"
  [obj_vaild] -> Switch4/2
  Bus Creator2/1 -> Switch4/3
  Switch4/1 -> cipv1/1
  Constant3/1 -> Bus Creator2/1  "MRR_ObjID"
  Constant2/1 -> Bus Creator2/2  "MRR_ObjDistX"
  Constant4/1 -> Bus Creator2/3  "MRR_ObjDistY"
  Constant5/1 -> Bus Creator2/4  "MRR_ObjRelVelX"
  Constant6/1 -> Bus Creator2/5  "MRR_ObjRelVelY"
  Constant7/1 -> Bus Creator2/6  "MRR_ObjType"
  Constant8/1 -> Bus Creator2/7  "MRR_ObjUpdFlg"
  Constant9/1 -> Bus Creator2/8  "obj_vaild"
  Constant10/1 -> Bus Creator2/9  "untracktime"
  IPM_obj/1 -> [IPM_obj]
  MRR_ObjFusionSig/1 -> [MRR_ObjFusionSig]
  MRR_ObjFusionCamID/1 -> [MRR_ObjFusionCamID]
  MRR_ObjType/1 -> [MRR_ObjType]
  [MRR_ObjType] -> Selector5/1
  MATLAB Function/1(y) -> Selector7/2
  Selector5/1 -> MATLAB Function/1(mrr_type)
  Selector10/1 -> MATLAB Function/4(hasCamera)
  [MRR_ObjFusionSig] -> Selector10/1
  [CIPV_index1] -> Selector8/2
  [CIPV_index1] -> Selector10/2
  Selector8/1 -> MATLAB Function/2(ipm_id)
  [MRR_ObjFusionCamID] -> Selector8/1
  [IPM_obj] -> MATLAB Function/3(ipm_obj)
  [MRR_ObjFusionCamID] -> Selector9/1
  [CIPV_index1] -> Selector9/2
  Selector9/1 -> Bus Creator1/10  "MRR_ObjFusionCamID"
  [CIPV_index1] -> Selector11/2
  [MRR_ObjFusionSig] -> Selector11/1
  Selector11/1 -> Bus Creator1/11  "MRR_ObjFusionSig"
  Constant11/1 -> Bus Creator2/10  "MRR_ObjFusionCamID"
  Constant12/1 -> Bus Creator2/11  "MRR_ObjFusionSig"

== system ALL_JP360_DBW_V6_5_1103/CIPV1/Obstacle selection/Subsystem1/If Action Subsystem ==
  In1 : Inport
  Action Port : ActionPort  ActionPortLabel=if(u1 < 0)
  Out1 : Outport
  wires:
  In1/1 -> Out1/1

== system ALL_JP360_DBW_V6_5_1103/CIPV1/Obstacle selection/Subsystem1/If Action Subsystem1 ==
  now_cipv1 : Inport
  last_cipv1 : Inport  Port=2
  Action Port : ActionPort  ActionPortLabel=elseif( u3>0)
  Bus Selector : BusSelector  OutputSignals=MRR_ObjDistX
  Bus Selector1 : BusSelector  OutputSignals=MRR_ObjDistX
  Constant2 : Constant  OutDataTypeStr=single
  GreaterThanOrEqual1 : RelationalOperator  OutDataTypeStr=boolean  RndMeth=Simplest  InputSameDT=off
  Plus1 : Sum  Inputs=+-
  Switch5 : Switch  Criteria=u2 > Threshold  SaturateOnIntegerOverflow=off  InputSameDT=off
  Out1 : Outport
  wires:
  now_cipv1/1 -> [now_cipv1]
  last_cipv1/1 -> [last_cipv1]
  [now_cipv1] -> Bus Selector/1
  [last_cipv1] -> Bus Selector1/1
  GreaterThanOrEqual1/1 -> Switch5/2
  Constant2/1 -> GreaterThanOrEqual1/2
  Plus1/1 -> GreaterThanOrEqual1/1
  Bus Selector/1 -> Plus1/1  "<MRR_ObjDistX>"
  Bus Selector1/1 -> Plus1/2  "<MRR_ObjDistX>"
  [now_cipv1] -> Switch5/3
  Switch5/1 -> Out1/1
  [last_cipv1] -> Switch5/1

== system ALL_JP360_DBW_V6_5_1103/CIPV1/Obstacle selection/Subsystem1/If Action Subsystem2 ==
  last_cipv1 : Inport
  IPM_Obj : Inport  Port=2
  Action Port : ActionPort  ActionPortLabel=else
  Bus Creator2 : BusCreator  Inputs=MRR_ObjID,MRR_ObjDistX,MRR_ObjDistY,MRR_ObjRelVelX,MRR_ObjRelVelY,MRR_ObjType,MRR_ObjUpdFlg,obj_vaild,untracktime,MRR_ObjFusionCamID,MRR_ObjFusionSig
  Bus Selector : BusSelector  OutputSignals=MRR_ObjDistX,untracktime,MRR_ObjFusionCamID,MRR_ObjFusionSig,MRR_ObjID,MRR_ObjDistX,MRR_ObjDistY,MRR_ObjRelVelX,MRR_ObjRelVelY,MRR_ObjType,MRR_ObjUpdFlg,obj_vaild
  MATLAB Function : MATLAB Function  TreatAsAtomicUnit=on
  Switch : Switch  Criteria=u2 > Threshold  Threshold=9  SaturateOnIntegerOverflow=off  InputSameDT=off
  Out1 : Outport
  wires:
  last_cipv1/1 -> [last_cipv1]
  IPM_Obj/1 -> [IPM_Obj]
  [last_cipv1] -> Bus Selector/1
  Bus Selector/1 -> [MRR_ObjDisstX]  "<MRR_ObjDistX>"
  Bus Selector/2 -> [untracktime]  "<untracktime>"
  Bus Selector/3 -> [MRR_ObjFusionCamID]  "<MRR_ObjFusionCamID>"
  Bus Selector/4 -> [MRR_ObjFusionSig]  "<MRR_ObjFusionSig>"
  [MRR_ObjDisstX] -> Switch/2
  [last_cipv1] -> Switch/1
  [IPM_Obj] -> MATLAB Function/1(IPM_Obj)
  [MRR_ObjFusionCamID] -> MATLAB Function/2(last_cipv1_MRR_ObjFusionCamID)
  [MRR_ObjFusionSig] -> MATLAB Function/3(last_cipv1_MRR_ObjFusionSig)
  Switch/1 -> Out1/1
  MATLAB Function/11(MRR_ObjFusionSig) -> Bus Creator2/11  "MRR_ObjFusionSig"
  MATLAB Function/10(MRR_ObjFusionCamID) -> Bus Creator2/10  "MRR_ObjFusionCamID"
  MATLAB Function/7(MRR_ObjUpdFlg) -> Bus Creator2/7  "MRR_ObjUpdFlg"
  MATLAB Function/8(obj_vaild) -> Bus Creator2/8  "obj_vaild"
  MATLAB Function/2(MRR_ObjDistX) -> Bus Creator2/2  "MRR_ObjDistX"
  MATLAB Function/9(untracktime) -> Bus Creator2/9  "untracktime"
  MATLAB Function/6(MRR_ObjType) -> Bus Creator2/6  "MRR_ObjType"
  MATLAB Function/1(MRR_ObjID) -> Bus Creator2/1  "MRR_ObjID"
  MATLAB Function/4(MRR_ObjRelVelX) -> Bus Creator2/4  "MRR_ObjRelVelX"
  MATLAB Function/5(MRR_ObjRelVelY) -> Bus Creator2/5  "MRR_ObjRelVelY"
  MATLAB Function/3(MRR_ObjDistY) -> Bus Creator2/3  "MRR_ObjDistY"
  Bus Selector/5 -> [MRR_ObjID]  "<MRR_ObjID>"
  Bus Selector/6 -> [MRR_ObjDistX]  "<MRR_ObjDistX>"
  Bus Selector/7 -> [MRR_ObjDistY]  "<MRR_ObjDistY>"
  Bus Selector/8 -> [MRR_ObjRelVelX]  "<MRR_ObjRelVelX>"
  Bus Selector/9 -> [MRR_ObjRelVelY]  "<MRR_ObjRelVelY>"
  Bus Selector/10 -> [MRR_ObjType]  "<MRR_ObjType>"
  Bus Selector/11 -> [MRR_ObjUpdFlg]  "<MRR_ObjUpdFlg>"
  Bus Selector/12 -> [obj_vaild]  "<obj_vaild>"
  [MRR_ObjID] -> MATLAB Function/4(last_cipv1_MRR_ObjID)
  [MRR_ObjDistX] -> MATLAB Function/5(last_cipv1_MRR_ObjDistX)
  [MRR_ObjDistY] -> MATLAB Function/6(last_cipv1_MRR_ObjDistY)
  [MRR_ObjRelVelX] -> MATLAB Function/7(last_cipv1_MRR_ObjRelVelX)
  [MRR_ObjRelVelY] -> MATLAB Function/8(last_cipv1_MRR_ObjRelVelY)
  [MRR_ObjType] -> MATLAB Function/9(last_cipv1_MRR_ObjType)
  [MRR_ObjUpdFlg] -> MATLAB Function/10(last_cipv1_MRR_ObjUpdFlg)
  [obj_vaild] -> MATLAB Function/11(last_cipv1_obj_vaild)
  [untracktime] -> MATLAB Function/12(last_cipv1_untracktime)
  Bus Creator2/1 -> Switch/3

== system ALL_JP360_DBW_V6_5_1103/CIPV1/Obstacle selection/Subsystem1/If Action Subsystem3 ==
  In1 : Inport
  Action Port : ActionPort  ActionPortLabel=elseif(u2>10)
  Out1 : Outport
  wires:
  In1/1 -> Out1/1

== system ALL_JP360_DBW_V6_5_1103/CIPV1/filter/filter lanes/get obj line y ==
  <IPM_Line01_C0> : Inport
  <IPM_Line01_C1> : Inport  Port=2
  <IPM_Line01_C2> : Inport  Port=3
  <IPM_Line01_C3> : Inport  Port=4
  objs_y : Inport  Port=5
  Constant : Constant  Value=1/2  OutDataTypeStr=single
  Constant1 : Constant  Value=1/6  OutDataTypeStr=single
  Plus : Sum  Inputs=++++
  Product1 : Product  Inputs=3
  Product2 : Product
  Product3 : Product  Inputs=3
  Product4 : Product
  Product5 : Product
  line_y : Outport
  wires:
  <IPM_Line01_C3>/1 -> Product3/2
  Constant/1 -> Product1/1
  Product2/1 -> Plus/2
  Product1/1 -> Plus/3
  Product3/1 -> Plus/4
  Constant1/1 -> Product3/1
  <IPM_Line01_C0>/1 -> Plus/1
  <IPM_Line01_C1>/1 -> Product2/1
  Plus/1 -> line_y/1
  <IPM_Line01_C2>/1 -> Product1/2
  objs_y/1 -> [objs_y]
  [objs_y] -> Product2/2
  [objs_y] -> Product4/1
  [objs_y] -> Product4/2
  Product4/1 -> [objs_y2]
  [objs_y2] -> Product1/3
  [objs_y2] -> Product5/1
  [objs_y] -> Product5/2
  Product5/1 -> [objs_y3]
  [objs_y3] -> Product3/3

== system ALL_JP360_DBW_V6_5_1103/CIPV1/filter/filter lanes/get obj line y1 ==
  <IPM_Line01_C0> : Inport
  <IPM_Line01_C1> : Inport  Port=2
  <IPM_Line01_C2> : Inport  Port=3
  <IPM_Line01_C3> : Inport  Port=4
  objs_y : Inport  Port=5
  Constant : Constant  Value=1/2  OutDataTypeStr=single
  Constant1 : Constant  Value=1/6  OutDataTypeStr=single
  Plus : Sum  Inputs=++++
  Product1 : Product  Inputs=3
  Product2 : Product
  Product3 : Product  Inputs=3
  Product4 : Product
  Product5 : Product
  line_y : Outport
  wires:
  <IPM_Line01_C3>/1 -> Product3/2
  Constant/1 -> Product1/1
  Product2/1 -> Plus/2
  Product1/1 -> Plus/3
  Product3/1 -> Plus/4
  Constant1/1 -> Product3/1
  <IPM_Line01_C0>/1 -> Plus/1
  <IPM_Line01_C1>/1 -> Product2/1
  Plus/1 -> line_y/1
  <IPM_Line01_C2>/1 -> Product1/2
  objs_y/1 -> [objs_y]
  [objs_y] -> Product2/2
  [objs_y] -> Product4/1
  [objs_y] -> Product4/2
  Product4/1 -> [objs_y2]
  [objs_y2] -> Product1/3
  [objs_y2] -> Product5/1
  [objs_y] -> Product5/2
  Product5/1 -> [objs_y3]
  [objs_y3] -> Product3/3

== system ALL_JP360_DBW_V6_5_1103/LKA_Control/LKA_Cal/ErrorCal/LatErrCal2 ==
  note: y1
  CenterLineCoeff : Inport
  VehPreviewPose : Inport  Port=2
  Abs : Abs  SaturateOnIntegerOverflow=off
  Add : Sum  Inputs=++++
  Add1 : Sum  Inputs=+-
  Constant : Constant  Value=2  OutDataTypeStr=single
  Constant1 : Constant  Value=3  OutDataTypeStr=single
  Constant2 : Constant  Value=0  OutDataTypeStr=single
  Demux : Demux
  Demux1 : Demux  Outputs=3
  Gain : Gain  Gain=1/2
  Gain1 : Gain  Gain=1/8
  Math Function : Math  Operator=pow
  Math Function1 : Math  Operator=pow
  Product : Product
  Product1 : Product
  Product2 : Product
  Relay : Relay  OnSwitchValue=0.001  OffSwitchValue=0.0005
  Switch : Switch  Criteria=u2 ~= 0  SaturateOnIntegerOverflow=off  InputSameDT=off
  To Workspace : ToWorkspace  VariableName=C3_status  SaveFormat=Structure With Time  SampleTime=-1
  theta : Terminator
  LatErr : Outport
  wires:
  CenterLineCoeff/1 -> Demux/1
  VehPreviewPose/1 -> Demux1/1
  Demux/1 -> Add/1
  Demux/2 -> Product/1
  Demux1/1 -> theta/1
  Demux1/2 -> Math Function1/1, Math Function/1, Product/2  "x1"
  Product/1 -> Add/2
  Constant/1 -> Math Function/2
  Demux/3 -> Abs/1, Gain/1
  Math Function/1 -> Product1/2
  Constant1/1 -> Math Function1/2
  Demux/4 -> Gain1/1
  Math Function1/1 -> Product2/2
  Add/1 -> Add1/1
  Demux1/3 -> Add1/2
  Add1/1 -> LatErr/1
  Gain/1 -> Product1/1
  Gain1/1 -> Product2/1
  Relay/1 -> To Workspace/1, Switch/2
  Constant2/1 -> Switch/3
  Switch/1 -> Add/4
  Product2/1 -> Switch/1
  Abs/1 -> Relay/1
  Product1/1 -> Add/3

== system ALL_JP360_DBW_V6_5_1103/LKA_Control/LKA_Cal/ErrorCal/VehiclePosePreview1 ==
  Input : Inport
  SAS_SteerWheelAngle : Inport  Port=2
  PreviewTime : Inport  Port=3
  Cos1 : Trigonometry  Operator=cos
  Divide1 : Product  Inputs=*/
  Gain3 : Gain  Gain=1/17.2
  Gain4 : Gain  Gain=1/3.6
  Gain5 : Gain  Gain=0.5  ParamDataTypeStr=single
  L-轴距1 : Constant  Value=3.27  OutDataTypeStr=single
  Product3 : Product  Inputs=3
  Product4 : Product  Inputs=3
  Product5 : Product  Inputs=3
  Sin1 : Trigonometry
  tan1 : Trigonometry  Operator=tan
  theta/varphi : Outport  OutDataTypeStr=single
  x1 : Outport  Port=2  OutDataTypeStr=single
  y1 : Outport  Port=3  OutDataTypeStr=single
  wires:
  Gain4/1 -> Product5/1, Product4/2, Product3/1
  Cos1/1 -> Product4/1
  Gain3/1 -> Gain5/1, tan1/1
  Gain5/1 -> Sin1/1, Cos1/1
  L-轴距1/1 -> Divide1/2
  Sin1/1 -> Product5/3
  Product3/1 -> Divide1/1
  tan1/1 -> Product3/3
  Divide1/1 -> theta/varphi/1
  Product4/1 -> x1/1
  Product5/1 -> y1/1
  Input/1 -> Gain4/1
  PreviewTime/1 -> Product5/2, Product4/3, Product3/2
  SAS_SteerWheelAngle/1 -> Gain3/1

== system ALL_JP360_DBW_V6_5_1103/button/ACCset/ACC_button/Subsystem1 ==
  speedout : Inport
  Chart : Stateflow chart  TreatAsAtomicUnit=on
  Chart10 : Stateflow chart  TreatAsAtomicUnit=on
  Constant4 : Constant  Value=0  OutDataTypeStr=boolean  SampleTime=0.01
  Constant5 : Constant  OutDataTypeStr=uint16  SampleTime=0.01
  Constant6 : Constant  OutDataTypeStr=boolean  SampleTime=0.01
  Data Type Conversion : DataTypeConversion  OutDataTypeStr=single  SaturateOnIntegerOverflow=off  RndMeth=Floor
  Data Type Conversion2 : DataTypeConversion  OutDataTypeStr=double  SaturateOnIntegerOverflow=off  RndMeth=Floor
  Delay : Delay
  Hit Crossing : HitCross  HitCrossingOffset=1  HitCrossingDirection=falling  ZeroCross=off
  OR6 : Logic  Operator=OR  IconShape=distinctive  AllPortsSameDT=off  OutDataTypeStr=boolean
  Product2 : Product
  Scope : Scope  NumInputPorts=2
  Switch4 : Switch  Criteria=u2 > Threshold  Threshold=85  SaturateOnIntegerOverflow=off  InputSameDT=off
  Out1 : Outport
  wires:
  Constant6/1 -> Switch4/1
  Constant4/1 -> Switch4/3
  Chart10/1(y) -> Scope/2, Delay/1
  Chart/1(y) -> Data Type Conversion/1, Scope/1, Switch4/2
  Data Type Conversion2/1 -> Hit Crossing/1
  OR6/1 -> Product2/2
  Switch4/1 -> OR6/1
  speedout/1 -> Chart/2(u1), Data Type Conversion2/1
  Hit Crossing/1 -> OR6/2
  Delay/1 -> Product2/1
  Constant5/1 -> Chart/1(t)
  Product2/1 -> Out1/1
  Data Type Conversion/1 -> Chart10/1(u1)

== system ALL_JP360_DBW_V6_5_1103/button/ACCset/ACC_button/Subsystem2 ==
  speedout : Inport
  Chart : Stateflow chart  TreatAsAtomicUnit=on
  Chart10 : Stateflow chart  TreatAsAtomicUnit=on
  Constant4 : Constant  Value=0  OutDataTypeStr=boolean  SampleTime=0.01
  Constant5 : Constant  OutDataTypeStr=uint16  SampleTime=0.01
  Constant6 : Constant  OutDataTypeStr=boolean  SampleTime=0.01
  Data Type Conversion2 : DataTypeConversion  OutDataTypeStr=double  SaturateOnIntegerOverflow=off  RndMeth=Floor
  Delay : Delay
  Hit Crossing : HitCross  HitCrossingOffset=1  HitCrossingDirection=falling  ZeroCross=off
  OR6 : Logic  Operator=OR  IconShape=distinctive  AllPortsSameDT=off  OutDataTypeStr=boolean
  Product2 : Product
  Switch4 : Switch  Criteria=u2 > Threshold  Threshold=85  SaturateOnIntegerOverflow=off  InputSameDT=off
  Out1 : Outport
  wires:
  Product2/1 -> Out1/1
  Constant5/1 -> Chart/1(t)
  Delay/1 -> Product2/1
  Hit Crossing/1 -> OR6/2
  speedout/1 -> Data Type Conversion2/1, Chart/2(u1)
  Switch4/1 -> OR6/1
  OR6/1 -> Product2/2
  Data Type Conversion2/1 -> Hit Crossing/1
  Chart/1(y) -> Chart10/1(u1), Switch4/2
  Chart10/1(y) -> Delay/1
  Constant4/1 -> Switch4/3
  Constant6/1 -> Switch4/1

== system ALL_JP360_DBW_V6_5_1103/button/ACCset/ACC_button/Subsystem3 ==
  speedout : Inport
  Chart : Stateflow chart  TreatAsAtomicUnit=on
  Chart10 : Stateflow chart  TreatAsAtomicUnit=on
  Constant4 : Constant  Value=0  OutDataTypeStr=boolean  SampleTime=0.01
  Constant5 : Constant  OutDataTypeStr=uint16  SampleTime=0.01
  Constant6 : Constant  OutDataTypeStr=boolean  SampleTime=0.01
  Data Type Conversion : DataTypeConversion  OutDataTypeStr=single  SaturateOnIntegerOverflow=off  RndMeth=Floor
  Data Type Conversion2 : DataTypeConversion  OutDataTypeStr=double  SaturateOnIntegerOverflow=off  RndMeth=Floor
  Delay : Delay
  Hit Crossing : HitCross  HitCrossingOffset=1  HitCrossingDirection=falling  ZeroCross=off
  OR6 : Logic  Operator=OR  IconShape=distinctive  AllPortsSameDT=off  OutDataTypeStr=boolean
  Product2 : Product
  Scope : Scope  NumInputPorts=2
  Switch4 : Switch  Criteria=u2 > Threshold  Threshold=85  SaturateOnIntegerOverflow=off  InputSameDT=off
  Out1 : Outport
  wires:
  Data Type Conversion/1 -> Chart10/1(u1)
  Product2/1 -> Out1/1
  Constant5/1 -> Chart/1(t)
  Delay/1 -> Product2/1
  Hit Crossing/1 -> OR6/2
  speedout/1 -> Data Type Conversion2/1, Chart/2(u1)
  Switch4/1 -> OR6/1
  OR6/1 -> Product2/2
  Data Type Conversion2/1 -> Hit Crossing/1
  Chart/1(y) -> Switch4/2, Scope/1, Data Type Conversion/1
  Chart10/1(y) -> Delay/1, Scope/2
  Constant4/1 -> Switch4/3
  Constant6/1 -> Switch4/1

== system ALL_JP360_DBW_V6_5_1103/button/ACCset/ACC_button/Subsystem4 ==
  speedout1 : Inport
  Chart1 : Stateflow chart  TreatAsAtomicUnit=on
  Chart2 : Stateflow chart  TreatAsAtomicUnit=on
  Constant1 : Constant  OutDataTypeStr=uint16  SampleTime=0.01
  Product1 : Product
  Saturation1 : Saturate  UpperLimit=50  LowerLimit=0  OutDataTypeStr=uint16
  Out1 : Outport
  wires:
  speedout1/1 -> Product1/2, Chart1/2(u1)
  Constant1/1 -> Chart1/1(t)
  Chart1/1(y) -> Saturation1/1
  Chart2/1(y) -> Product1/1
  Product1/1 -> Out1/1
  Saturation1/1 -> Chart2/1(u1)
